simulink model "ava1"  (R2017b)
settings: Solver=VariableStepAuto  StartTime=0.0  StopTime=10.0  RelTol=1e-3
model workspace (MAT data in the model file):
  gnc_Q_EKF = [5.72003821599e-08 5.72003821599e-08 5.72003821599e-08 6.11350238322e-12 6.11350238322e-12 6.11350238322e-12 2.33611111111e-05 2.33611111111e-05 2.33611111111e-05 4.70596e-05 4.70596e-05 4.70596e-05 5.1480343944e-07 5.72003821599e-08 5.72003821599e-08 5.5021521449e-11 6.11350238322e-12 6.11350238322e-12]
  gnc_R_gps_pos = [400  0  0; 0  400  0; 0  0  400]
  gnc_R_gps_vel = [0.0016  0  0; 0  0.0016  0; 0  0  0.0016]
  gnc_R_mag = [0.002025  0  0; 0  0.002025  0; 0  0  0.002025]
settings Model: Creator=hbourbou  LastModifiedBy=hbourbou

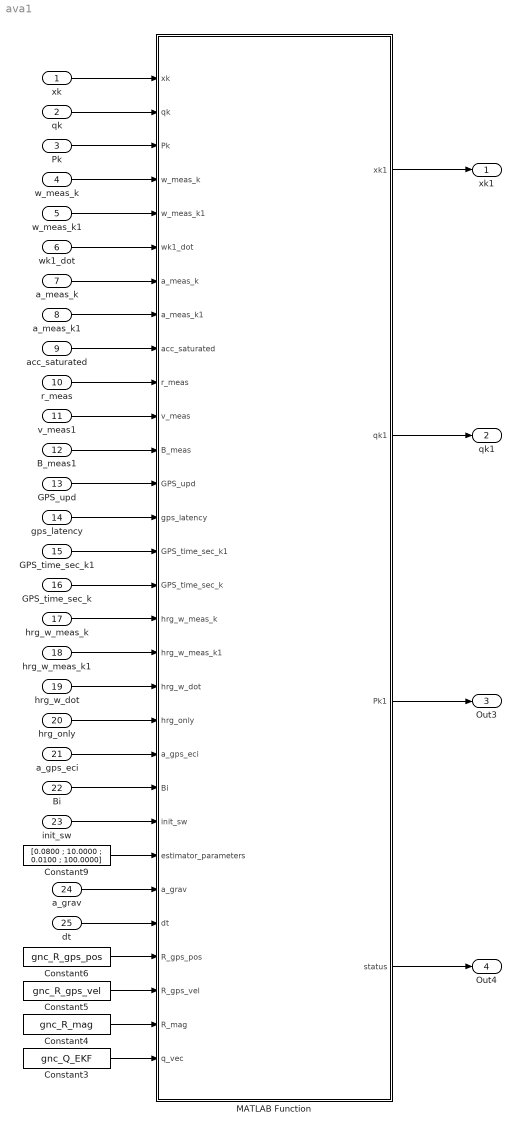
== system ava1 ==
  xk : Inport  PortDimensions=18
  qk : Inport  Port=2  PortDimensions=4
  Pk : Inport  Port=3  PortDimensions=[18, 18]
  w_meas_k : Inport  Port=4  PortDimensions=3
  w_meas_k1 : Inport  Port=5  PortDimensions=3
  wk1_dot : Inport  Port=6  PortDimensions=3
  a_meas_k : Inport  Port=7  PortDimensions=3
  a_meas_k1 : Inport  Port=8  PortDimensions=3
  acc_saturated : Inport  Port=9
  r_meas : Inport  Port=10  PortDimensions=3
  v_meas1 : Inport  Port=11  PortDimensions=3
  B_meas1 : Inport  Port=12  PortDimensions=3
  GPS_upd : Inport  Port=13
  gps_latency : Inport  Port=14
  GPS_time_sec_k1 : Inport  Port=15
  GPS_time_sec_k : Inport  Port=16
  hrg_w_meas_k : Inport  Port=17  PortDimensions=3
  hrg_w_meas_k1 : Inport  Port=18  PortDimensions=3
  hrg_w_dot : Inport  Port=19  PortDimensions=3
  hrg_only : Inport  Port=20
  a_gps_eci : Inport  Port=21  PortDimensions=3
  Bi : Inport  Port=22  PortDimensions=3
  init_sw : Inport  Port=23  OutDataTypeStr=boolean
  a_grav : Inport  Port=24  PortDimensions=3
  dt : Inport  Port=25
  Constant3 : Constant  Value=gnc_Q_EKF
  Constant4 : Constant  Value=gnc_R_mag
  Constant5 : Constant  Value=gnc_R_gps_vel
  Constant6 : Constant  Value=gnc_R_gps_pos
  Constant9 : Constant  Value=|
      | [0.0800
      | ;   10.0000
      | ;    0.0100
      | ;  100.0000]
  MATLAB Function : MATLAB Function  TreatAsAtomicUnit=on
  xk1 : Outport
  qk1 : Outport  Port=2
  Out3 : Outport  Port=3
  Out4 : Outport  Port=4
  wires:
  MATLAB Function/1(xk1) -> xk1/1
  MATLAB Function/2(qk1) -> qk1/1
  MATLAB Function/3(Pk1) -> Out3/1
  MATLAB Function/4(status) -> Out4/1
  xk/1 -> MATLAB Function/1(xk)
  qk/1 -> MATLAB Function/2(qk)
  Pk/1 -> MATLAB Function/3(Pk)
  w_meas_k/1 -> MATLAB Function/4(w_meas_k)
  w_meas_k1/1 -> MATLAB Function/5(w_meas_k1)
  wk1_dot/1 -> MATLAB Function/6(wk1_dot)
  a_meas_k/1 -> MATLAB Function/7(a_meas_k)
  a_meas_k1/1 -> MATLAB Function/8(a_meas_k1)
  acc_saturated/1 -> MATLAB Function/9(acc_saturated)
  r_meas/1 -> MATLAB Function/10(r_meas)
  v_meas1/1 -> MATLAB Function/11(v_meas)
  B_meas1/1 -> MATLAB Function/12(B_meas)
  GPS_upd/1 -> MATLAB Function/13(GPS_upd)
  gps_latency/1 -> MATLAB Function/14(gps_latency)
  GPS_time_sec_k1/1 -> MATLAB Function/15(GPS_time_sec_k1)
  GPS_time_sec_k/1 -> MATLAB Function/16(GPS_time_sec_k)
  hrg_w_meas_k/1 -> MATLAB Function/17(hrg_w_meas_k)
  hrg_w_meas_k1/1 -> MATLAB Function/18(hrg_w_meas_k1)
  hrg_w_dot/1 -> MATLAB Function/19(hrg_w_dot)
  hrg_only/1 -> MATLAB Function/20(hrg_only)
  a_gps_eci/1 -> MATLAB Function/21(a_gps_eci)
  Bi/1 -> MATLAB Function/22(Bi)
  init_sw/1 -> MATLAB Function/23(init_sw)
  Constant9/1 -> MATLAB Function/24(estimator_parameters)
  a_grav/1 -> MATLAB Function/25(a_grav)
  dt/1 -> MATLAB Function/26(dt)
  Constant6/1 -> MATLAB Function/27(R_gps_pos)
  Constant5/1 -> MATLAB Function/28(R_gps_vel)
  Constant4/1 -> MATLAB Function/29(R_mag)
  Constant3/1 -> MATLAB Function/30(q_vec)

== matlab function ava1/MATLAB Function ==
  data: xk input size=18; qk input size=4; xk1 output size=18; qk1 output size=4; Pk input; w_meas_k input; w_meas_k1 input; wk1_dot input; a_meas_k input; a_meas_k1 input; acc_saturated input; r_meas input; v_meas input; B_meas input; GPS_upd input; gps_latency input; GPS_time_sec_k1 input; GPS_time_sec_k input; hrg_w_meas_k input; hrg_w_meas_k1 input; hrg_w_dot input; hrg_only input; a_gps_eci input; Bi input; init_sw input; estimator_parameters input; a_grav input; dt input; R_gps_pos input; R_gps_vel input; R_mag input; q_vec input; Pk1 output; status output
function [xk1,qk1,Pk1,    status]   = INS_GPS_EKF_swords(xk,qk,Pk,w_meas_k,w_meas_k1,wk1_dot,a_meas_k,a_meas_k1,acc_saturated, r_meas,...
    v_meas, B_meas,GPS_upd,gps_latency,GPS_time_sec_k1, GPS_time_sec_k, hrg_w_meas_k, hrg_w_meas_k1, hrg_w_dot, hrg_only,a_gps_eci,Bi,init_sw,... 
    estimator_parameters, a_grav, dt, R_gps_pos,R_gps_vel,R_mag, q_vec ) 

%%%%
%#codegen

a_bar_inertial=[0 0 0]';
err=0; %Error code : 1-negetive S,
a_e=[0 0 0]';
mu = 3.9860e+14; %398600*1000*1000*1000;
valid_GPS_meas=(GPS_upd == 1)&&(GPS_time_sec_k > 0)&&(GPS_time_sec_k1 > GPS_time_sec_k + dt-0.01);
valid_Mag_meas=norm(Bi)>0 && norm(B_meas)>0;
valid_Acc_meas=norm(a_meas_k)>0.5 && norm(a_meas_k1)>0.5;
scale_flag=single([0 0 0]');dscaler=[0.0 0.0 0.0]';scaler=zeros(3,3);diagscaler=diag(scaler);

status=0; %Status bit
          %8:reserved(MSB)
          %7:DIVERGING
          %6:bias convergency
          %5:attitude convergency
          %4:transition convergency
          %3:magnetometer measurement available
          %2:GPS available
          %1:initilized



if hrg_only
    wk =  hrg_w_meas_k;
    wk1 = hrg_w_meas_k1;
    wk1_dot=hrg_w_dot;
else
    wk = w_meas_k;
    wk1 = w_meas_k1;
end

ak = a_meas_k;
ak1 = a_meas_k1;
a_bar= .5*a_meas_k + .5*a_meas_k1;

rk = xk(4:6);
vk = xk(7:9);    

if init_sw ~= 0 || norm(a_grav)==0
    xk1 = xk;
    Pk1 = Pk;
    qk1 = qk;    
    return;
end

%Initilization done
status = bitor(status, bin2dec('00000001')); 

%(18by1)vector q ->(18by18)matrix Q
Q=zeros(18,18);
for i=1:18
    Q(i,i)=q_vec(i);
end

%%%%%%%%%%% (1) propagate state %%%%%%%%%%%
%acclerometer screening during free fall
flag_freefall=0;
if (norm(ak1)<8 && norm(ak)<8) 
    flag_freefall=1;
end

%propagate attitude
%1st order
wbar = (wk1 + wk)/2; %wbar_hrg=(hrg_wk+hrg_wk1)/2;
qk1 = (eye(4) + dt/2*Omega(wbar) + 1/48*(Omega(wk1)*Omega(wk) - Omega(wk)*Omega(wk1))*dt^2)*qk;
%2nd order term
qk1 = qk1+.5*(.5^2*Omega(wbar)*Omega(wbar)*dt^2)*qk;

%%% still tunning
R_i2b_k1_delay=eye(3,3);
%%%%%%%%TEST%%%%%%%%%%%%%%%%%%%%%%%%%%%%%%%%%%%%%%%%%%%%%%%%%%%%%%%
if 1 %Preparation for compensating magnetometer delay, gps_latency ALWAYS.
    %if norm(wbar)>pi %delay compensation only high rate when w >180 degree/second.
    %compensating mag delay    
    %Preparation for compensating magnetometer delay, gps_latency
    
    qk1_mag=(eye(4) + (gps_latency)/2*Omega(wbar))*[0 0 0 1]';        
    R_i2b_k1_delay= quat_to_dcm(qk1_mag);
end

%normalize
qk1_squared=sum(qk1.^2);
if qk1_squared ~=0
    qk1 = qk1/(sqrt(qk1_squared));
end

%prepare transition from B2I & I2B
R_i2b_k = quat_to_dcm(qk);    R_b2i_k = R_i2b_k';
R_i2b_k1 = quat_to_dcm(qk1);  R_b2i_k1 = R_i2b_k1';

%propagate position/velocity ECI
ak_inertial = R_b2i_k*ak + a_grav; %a_inertial = R_b2i_k*ak;
ak1_inertial = R_b2i_k1*ak1 + a_grav;

%%% use gps based ACC when acc bias is too big, saturated???
if (acc_saturated && norm(ak1)>100) 
    a_bar_inertial=a_gps_eci;
else
    a_bar_inertial=ak_inertial*.5+ak1_inertial*.5;
end
   
%integrate average (linear) accel to get velocity
if flag_freefall
    vk1 = vk + a_gps_eci *dt;%vk1 = vk + ak_inertial*dt;
else
    vk1 = vk + a_bar_inertial *dt;%vk1 = vk + ak_inertial*dt;
end
rk1 = rk + vk*dt; %rk1 = rk + vk*dt + (2*ak_inertial + ak1_inertial)/6*dt^2;
    
% if 0, %No sensor lag compensated, Measurement will not be modified w/ state for stability 
%     %propagate measurements 2 timesteps to account for gps_latency
%     %v_meas = v_meas + a_gps_eci*(gps_latency); 
%     v_meas = v_meas + (ak_inertial + ak1_inertial)/2*(gps_latency);
%     r_meas = r_meas + v_meas*(gps_latency);
%     %r_meas = r_meas + (2*ak_inertial + ak1_inertial)/6*(gps_latency)^2;
% end
    
%%%%%%%%%%% (2) propagate covariance %%%%%%%%%%%
% Coavairance of propagation is scaled up because state has only bias but no scaler
% TBD, estimate scale factor of gyro
%  Q~~[gyroNoise gyroDynamic AccNoise AccDynamic highRateNoise HighRateDynamics]
%W_dot based scaling not used
%w_dot_threshold = estimator_parameters(1);w_dot_scale = estimator_parameters(2);
w_threshold = estimator_parameters(3);w_scale =estimator_parameters(4);

%scale_flag=single(abs(wk1_dot)>w_dot_threshold & abs(wk1)>w_threshold); 
scale_flag=single( abs(wk1)>w_threshold); 
diag_scale_flag=diag(scale_flag);

scaler = eye(3)+ diag_scale_flag* diag(abs(wk1)*w_scale/10)^2;     
%%%%%TEST%%%%%%%%%%%%%%%%%%%%%%%%%%%%%%%%%%%%%%%%%%%%%%%%%%%%%%%%%%%%%
Q(16:18,16:18)=Q(16:18,16:18)*scaler;     %HRG bias dynamics covriance

if ~hrg_only     
     Q(4:6,4:6)=Q(4:6,4:6)*scaler;     
     dscaler=diag(double(scaler)); %to monitor the scale
     
     %scaler = eye(3)+diag_scale_flag *diag(abs(wk1)*w_scale/10 )^2;
     Q(1:3,1:3)=Q(1:3,1:3)*scaler;          
else
    %%%%%%%%%%%%%%%%%%%%%%%%%%%TEST%%%%%%%%%%%%%%%%%%%%%%%%%%%%%%%%%%
    Q(4:6,4:6)=Q(4:6,4:6)*scaler;         
    Q(13:15,13:15)=Q(13:15,13:15)*scaler;     %HRG bias dynamics covriance
    
end

%%%%%%%
%ACC bias dynamics Cov scaled by the velocity in body 
%Inertial Sensor Arrays – A Literature Review, John-Olof Nilsson and Isaac Skog
%if 0, %0 for SL-11 FIX   %%%%%%%%%DEBUG for 1!!!!!!!!!!!!!!!!!!!!!!!!!!!!!!!!!!!!!!!!!!!!!!!!!!!!! change into 0
%    v_b_k1=R_i2b_k1*vk1;
%    scaler = eye(3)+ diag_scale_flag *diag(abs(wk1)*w_scale/10 )^2; %for centripetal from acc location offset
%    scaler = scaler + diag(single(abs(v_b_k1)>100)) *diag(abs(v_b_k1)/100 )^2; %for gps velocity delay
%    Q(10:12,10:12)=Q(10:12,10:12)*scaler ;
%else    
    acc_location_error=0.05; %meter
    scaler_acc_bias = eye(3)+ diag(cross(wk1, cross(wk1,[1 1 1]'*acc_location_error)))^2; %for centrifugal from acc location offset
    scaler_acc_bias = scaler_acc_bias + diag(cross(wk1_dot,[1 1 1]'*acc_location_error))^2;       %for Euler Force from acc offset
    
    v_b_k1=R_i2b_k1*vk1;
    %%%TEST!!!!!!!!!!!!!!!!!!!!!!!!!!!!
    %scaler_acc_bias = scaler_acc_bias + diag(single(abs(v_b_k1)>100)) *diag(abs(v_b_k1)/100 )^2; %for gps velocity delay
    %%%%%%%%%%%%%%%%%%%%%%%%%%%%%%%%
    Q(10:12,10:12)=Q(10:12,10:12)*scaler_acc_bias ;
%end

%Acc Bias Noise covariance
%small cov makes the filter believe acc more and less GPS velocity.
%ACC meas error Cov VS spin Rate-might not related. but this seems to be
%the most reasonable way to scale uncertainty of ACC 
%for ACC varies from ~0.1g up to mor ethan 10 g+
%%%%%%%%%%%%%%%%%%%%%%%%%%%%%%%%%%%%%%%%%%%%%%%%%%%%%%%%%%%% TEST!!!
Q(7:9,7:9)=    Q(7:9,7:9)*scaler_acc_bias;
%Q(7:9,7:9)=    Q(7:9,7:9)*scaler_acc_bias*100 ; 

%scaler = eye(3)+ diag(single(abs(wk1)>0.1)) *diag(abs(wk1)/0.1 )^2;
%Q(7:9,7:9)=    Q(7:9,7:9)*scaler ;

%%%test ##
if flag_freefall %ACC is not used during freefall
    Q(7:9,7:9)=Q(7:9,7:9)*eye(3,3)*1000000;
    Q(10:12,10:12)=Q(10:12,10:12)*eye(3,3)*1000000;
end
%%%%%
%%%%%%%%%%%%%%%%%%%%%%%%%%%%%%%%%%%%%%%%%%%%%%%%%%%%%


%build STM, F x State, State = [ quaternion3 pos3 vel3 gyroi_bias3 acc_bias3 hrg_bias3]
F = zeros(18);
F(1:3,1:3) = -skew(wk);
if hrg_only   
    F(1:3,16:18) = -eye(3); %by hrg bias              
else
    F(1:3,10:12) = -eye(3); %by gyro bias
    %F(1:3,16:18) = -eye(3); %by hrg bias, .When gyro is used hrg isn't.
end

F(4:6,7:9) = eye(3);
F(7:9,1:3) = - R_b2i_k*skew(a_bar);    
F(7:9,4:6) = F_2body(mu,rk); %gravity sensitivity %use J2?
F(7:9,13:15) = -R_b2i_k;     %Velocity from accelerometer bias 

%%%%%%%%%%debugging These for ECEF<-> BODY
%F(7:9, 7:9)=-2*skew(wk);
%F(7:9, 4:6)= -(skew(wk)*skew(wk));
%%%


%noise covariance matrix %G x Q, Q =[gyroNoise gyroDynamic AccNoise AccDynamic highRateNoise HighRateDynamics]
G = zeros(18,18);
if hrg_only
    G(1,13)=-1.0;G(2,14)=-1.0;G(3,15)=-1.0; %hrg noise                  G(1:3,13:15) = -eye(3);  
else    
    G(1,1)=-1.0;G(2,2)=-1.0;G(3,3)=-1.0; %gyro noise G(1:3,1:3) = -eye(3);    
end
G(7:9,7:9) = -R_b2i_k;
G(10,4) =1.0;G(11, 5) =1.0;G(12,6) =1.0; %G(10:12,4:6) = eye(3);   %Gyro bias rate noise
G(13,10)=1.0;G(14,11) =1.0;G(15,12)=1.0; %G(13:15,10:12) = eye(3); %Accel bias
G(16,16)=1.0;G(17,17) =1.0;G(18,18)=1.0;%G(16:18, 16:18) = eye(3); %HRG bias rate noise 

%Matt's attmept to speed things up
Phi = eye(18) + F*dt + 0.5*F^2*dt^2;
Qd = G*Q*G'*dt;

%compute Phi and Qd in block form a la Crassidis paper
% A = [-F G*Q*G'; zeros(18) F'];
% B = eye(36) + A*dt + 0.5*A^2*dt^2;
% Phi = B(19:36,19:36)';
% Qd = Phi*B(1:18,19:36);

%propagate covariance
Pk1 = Phi*Pk*Phi' + Qd;

%%
%%%%%%%%%%% (3) compute Kalman gain %%%%%%%%%%%
%residual = meas - ref
%%%

H=zeros(0,18);R=zeros(0,0);r=zeros(0,1);
if valid_Mag_meas
    H_mag = skew(R_i2b_k1*Bi); %2*skew(R_i2b*Bi)?
    r_mag = R_i2b_k1_delay*B_meas - R_i2b_k1*Bi;
    H = [H_mag zeros(3) zeros(3) zeros(3) zeros(3) zeros(3)];
    if norm(a_bar_inertial)<1
        R_mag=R_mag/500;
    end
    R=  blkdiag(R_mag); 
    
    r=[r_mag];
end
if valid_GPS_meas        
    H=[H;zeros(3) eye(3) zeros(3) zeros(3) zeros(3) zeros(3);...
        zeros(3) zeros(3) eye(3) zeros(3) zeros(3) zeros(3)];
    position_uncertainty_scaler= eye(3)+ diag( (abs(v_meas)/400).^2);    
    R = blkdiag(R, R_gps_pos* position_uncertainty_scaler ,R_gps_vel);
    r_gps_pos = r_meas - rk1;
    r_gps_vel = v_meas - vk1; 
    r=[r;r_gps_pos;r_gps_vel]; 
end

if  ~hrg_only  %Additional eq for hrg bias est
    r_hrg=  (hrg_w_meas_k1+hrg_w_meas_k)/2-(wbar) ;
    H= [H;...          
         zeros(3,15) eye(3)];    
    R= blkdiag(R, 0.01^2*eye(3)); %1^2 gyro + hrg (=3^2 gyro) 0.05^2*eye(3)
    r= [r; r_hrg];
end

%high velocity where body axis is assumed to be aligned with GPS velocity
% if  norm(v_meas)>20   %attitude is already GOOD during this high velocity period
%     H_gps_vel= - 0.5*(R_b2i_k1*skew([-norm(vk1) 0 0]') + R_b2i_k*skew([-norm(vk) 0 0]'));    
%     r_gps_vel = v_meas-(R_b2i_k1*[-norm(vk1) 0 0]' +R_b2i_k*[-norm(vk) 0 0]')/2;
%     H= [H;...          
%         H_gps_vel zeros(3,15)];
%     R= blkdiag(R, 10^2*eye(3)); %
%     r= [r; r_gps_vel];
% end


%Pk matrix integrity check and bandading instead of crach on real time, 
% Not used for heavy calculation of eig
% if sum(eig(Pk1)<0)>0
%     err=1; %Will publish this out later
%     Pk1=Pk1/2+Pk1'/2;    
%     Pk1=Pk1+eye(18)*eps;
% end

%%
%%%%%%%%%%% (4) update state %%%%%%%%%%%
    
if valid_Mag_meas || valid_GPS_meas
    S = H*Pk1*H' + R;
    K = Pk1*H'/S;   %Kalman gain
    

    delta_x = K*r;
    
    %update quaternion    
    delq=.5 * delta_x(1:3,1);
    delQ=1/sqrt(1+sum(delq.^2))*[delq; 1]';    
    qk1=QuatProd(delQ)*qk1;   
    
    %update bias
    gyro_bias_k1 = xk(10:12) + delta_x(10:12,1);
    if valid_GPS_meas 
        accel_bias_k1 = xk(13:15) + delta_x(13:15,1);    
        %update position and velocity
        rk1 = rk1 + delta_x(4:6,1);
        vk1 = vk1 + delta_x(7:9,1);  
        status = bitor(status, bin2dec('00000010'));
    else 
        accel_bias_k1 = xk(13:15);
    end
    
    if acc_saturated
        accel_bias_k1(1) = xk(13); %For only body x-axis
    end
    
    hrg_bias_k1=xk(16:18)+ delta_x(16:18,1);    
    xk1 = [zeros(3,1);rk1;vk1;gyro_bias_k1;accel_bias_k1;hrg_bias_k1];
    
    if hrg_only
       xk1(10)=  xk(10); %bias scaled rapidely during high rotation
       xk1(11:12)=xk1(17:18);       
    else 
       xk1(17:18)=xk1(11:12);
    end

 
 %%
 %%%%%%%%%%% (5) update covariance %%%%%%%%%%%  
    Pk1 =(eye(18)-K*H)*Pk1*(eye(18)-K*H)'+K*R*K';
    
    if valid_Mag_meas, status = bitor(status, bin2dec('00000100'));end        
else
    xk1 = [zeros(3,1);rk1;vk1;xk(10:18)];
end

converging_transition =sum(diag(Pk1(4:9,4:9)));
converging_attitude =sum(diag(Pk1(1:3,1:3)));
converging_bias =sum(diag(Pk1(10:16,10:16)));
if converging_transition < 10 %Biggest part of covariance is of the position.    
    status = bitor(status, bin2dec('00001000'));
end
if converging_attitude < 20^(-3), %Biggest part of covariance is of the position.    
    status = bitor(status, bin2dec('00010000'));
end
if converging_bias < 0.6,
    status = bitor(status, bin2dec('00100000'));
end
if (sum(diag(Pk1))>1e7),  %Diverging, reset operation will require.
    status = bitor(status, bin2dec('01000000'));
end


end
%State = [ quaternion3 pos3 vel3 gyroi_bias3 acc_bias3 hrg_bias3]
% x_dot=fx +GQ
% f=[F11 0   0   F14 0 0;     G=[G11       0  0     0 G14 0 ] G11(gyro) or G14(hrg)=I
%    0   0   I   0   0 0;       [0         0 0      0 0   0
%    F31 F32 F33 0 F35 0;       [ 0        0 -R_b2i 0 0   0
%    0   0   0   0  0  0;       [0         I  0     0 0   0
%    0   0   0  0   0  0];      [0         0  0     0 I   0]
% Q =[gyroNoise gyroDynamic AccNoise AccDynamic highRateNoise HighRateDynamics]

function z=QuatProd(q)
z=[q(4)*eye(3)-skew(q(1:3)) q(1:3)';...
    -q(1:3)                  q(4)];
end
function Om = Omega(w)
Om = [0,w(3),-w(2),w(1);-w(3),0,w(1),w(2);w(2),-w(1),0,w(3);-w(1),-w(2),-w(3),0];
end

function xhat = skew(x)
% Computes the hat map, mapping a 3-vector into a 3X3 skew-symmetric matrix
xhat = [  0   -x(3)  x(2)
         x(3)   0   -x(1)
        -x(2)  x(1)  0];
end

function z = Xi(q)
z = [q(4)*eye(3) + skew(q(1:3));-q(1:3)'];
end

function F = F_2body(mu,r)
r_mag = norm(r);
rx = r(1);
ry = r(2);
rz = r(3);

r3 = r_mag*r_mag*r_mag;
r5 = r_mag*r_mag*r_mag*r_mag*r_mag;

F11 = -mu/r3 + 3*mu*rx^2/r5;
F12 = 3*mu*rx*ry/r5;
F13 = 3*mu*rx*rz/r5;
F22 = -mu/r3 + 3*mu*ry^2/r5;
F23 = 3*mu*ry*rz/r5;
F33 = -mu/r3 + 3*mu*rz^2/r5;

F = [F11 F12 F13; F12 F22 F23; F13 F23 F33];
end

function dcm = quat_to_dcm(q)
q1 = q(1);
q2 = q(2);
q3 = q(3);
q4 = q(4);

dcm = zeros(3,3);

dcm(1,1) = q1^2 - q2^2 - q3^2 + q4^2;
dcm(2,1) = 2 * ( q1*q2 - q3*q4 ) ;
dcm(3,1) = 2 * ( q1*q3 + q2*q4 ) ;
dcm(1,2) = 2 * ( q1*q2 + q3*q4 ) ;
dcm(2,2) = -q1^2 + q2^2 - q3^2 + q4^2;
dcm(3,2) = 2 * ( q2*q3 - q1*q4 ) ;
dcm(1,3) = 2 * ( q1*q3 - q2*q4 ) ;
dcm(2,3) = 2 * ( q2*q3 + q1*q4 );
dcm(3,3) = -q1^2 - q2^2 + q3^2 + q4^2;
end

function scaler = getScale(wk1, wk1_dot, diag_scale_flag,w_scale,w_dot_scale)
%w_dot_scale = estimator_parameters(2);
%w_scale =estimator_parameters(4);

scaler = eye(3)+ diag_scale_flag* diag(abs(wk1)*w_scale +...
    abs(wk1_dot*w_dot_scale))^2;
scaler_limit= 5*10^6;
scaler=(scaler>scaler_limit)*scaler_limit +diag(diag((scaler <=scaler_limit)));
end
%%%
% function a_grav = getGrav(r_meas,valid_GPS_meas,rk,mu)
% a_grav =zeros(3,1);
% if valid_GPS_meas, 
%     rk_norm =norm(r_meas);    
% else
%     rk_norm =norm(rk);    
% end
% if rk_norm>=0,
%     a_grav     =-mu*r_meas/(rk_norm^3);
% end
% end
